simulink model "astatism"  (Simulink 7.3)
settings: Solver=ode45  StartTime=0.0  StopTime=4  RelTol=1e-3
settings Model: Creator=Sainquake  LastModifiedBy=Sainquake

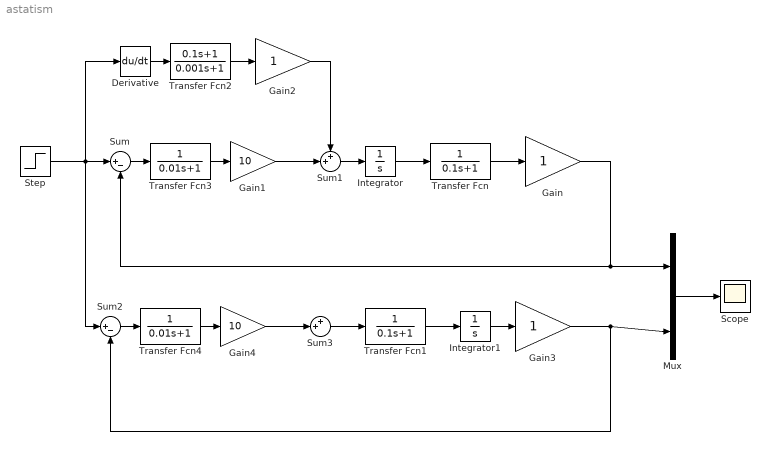
== system astatism ==
  Derivative : Derivative
  Gain : Gain  ParameterDataType=fixdt(1, 16)  ParameterScaling=2^0  OutDataType=fixdt(1, 16)  OutScaling=2^0
  Gain1 : Gain  Gain=10  ParameterDataType=fixdt(1, 16)  ParameterScaling=2^0  OutDataType=fixdt(1, 16)  OutScaling=2^0
  Gain2 : Gain  ParameterDataType=fixdt(1, 16)  ParameterScaling=2^0  OutDataType=fixdt(1, 16)  OutScaling=2^0
  Gain3 : Gain  ParameterDataType=fixdt(1, 16)  ParameterScaling=2^0  OutDataType=fixdt(1, 16)  OutScaling=2^0
  Gain4 : Gain  Gain=10  ParameterDataType=fixdt(1, 16)  ParameterScaling=2^0  OutDataType=fixdt(1, 16)  OutScaling=2^0
  Integrator : Integrator
  Integrator1 : Integrator
  Mux : Mux  Inputs=2
  Scope : Scope
  Step : Step  SampleTime=0
  Sum : Sum  Inputs=|+-  OutDataType=fixdt(1, 16)  OutScaling=2^0
  Sum1 : Sum  Inputs=++|  OutDataType=fixdt(1, 16)  OutScaling=2^0
  Sum2 : Sum  Inputs=|+-  OutDataType=fixdt(1, 16)  OutScaling=2^0
  Sum3 : Sum  Inputs=++|  OutDataType=fixdt(1, 16)  OutScaling=2^0
  Transfer Fcn : TransferFcn  Denominator=[0.1 1]
  Transfer Fcn1 : TransferFcn  Denominator=[0.1 1]
  Transfer Fcn2 : TransferFcn  Numerator=[0.1 1]  Denominator=[0.001 1]
  Transfer Fcn3 : TransferFcn  Denominator=[0.01 1]
  Transfer Fcn4 : TransferFcn  Denominator=[0.01 1]
  wires:
  Integrator/1 -> Transfer Fcn/1
  Gain/1 -> Sum/2, Mux/1
  Gain1/1 -> Sum1/2
  Sum/1 -> Transfer Fcn3/1
  Step/1 -> Sum/1, Derivative/1, Sum2/1
  Sum1/1 -> Integrator/1
  Gain2/1 -> Sum1/1
  Integrator1/1 -> Gain3/1
  Gain3/1 -> Sum2/2, Mux/2
  Gain4/1 -> Sum3/2
  Sum2/1 -> Transfer Fcn4/1
  Sum3/1 -> Transfer Fcn1/1
  Mux/1 -> Scope/1
  Transfer Fcn3/1 -> Gain1/1
  Transfer Fcn4/1 -> Gain4/1
  Transfer Fcn/1 -> Gain/1
  Transfer Fcn1/1 -> Integrator1/1
  Derivative/1 -> Transfer Fcn2/1
  Transfer Fcn2/1 -> Gain2/1
